simulink model "RealTimeMachine"  (R2021a)
settings: Solver=FixedStepDiscrete  StartTime=0.0  StopTime=Inf  FixedStep=TSampleRTM  MaxStep=1e-3  RelTol=1e-3  EnableMultiTasking=on
settings Model: SimulationMode=external  ExtModeTrigDuration=8  Creator=lu  LastModifiedBy=lu
settings SolverCC: AlgebraicLoopSolver=TrustRegion  AutoInsertRateTranBlk=on
settings OptimizationCC: DefaultUnderspecifiedDataType=single  PassReuseOutputArgsAs=Individual arguments  MaxStackSize=1024  DenormalBehavior=FlushToZero  EfficientTunableParamExpr=on
settings DebuggingCC: ParameterTunabilityLossMsg=error  SFMachineParentedDataDiag=warning
settings HardwareCC: ProdBitPerChar=16  ProdBitPerInt=16  ProdBitPerPointer=32  ProdBitPerSizeT=32  ProdBitPerPtrDiffT=32  ProdLargestAtomicInteger=Integer  ProdLargestAtomicFloat=None  ProdWordSize=16  ProdLongLongMode=on  ProdHWDeviceType=Texas Instruments->C2000
settings ModelReferenceCC: ModelReferenceNumInstancesAllowed=Single
settings SFSimCC: MATLABDynamicMemAlloc=off
settings RTWCC: SystemTargetFile=ert.tlc  HardwareBoard=TI Piccolo F28004x  GenCodeOnly=on  TemplateMakefile=ert_default_tmf  GenerateReport=on  Toolchain=Texas Instruments Code Composer Studio (C2000)  IncludeHyperlinkInReport=on  LaunchReport=on  GenerateTraceInfo=on  GenerateTraceReport=on  GenerateTraceReportSl=on  GenerateTraceReportSf=on  GenerateTraceReportEml=on  GenerateWebview=on  GenerateCodeMetricsReport=on
settings CodeAppCC: ForceParamTrailComments=on  IgnoreCustomStorageClasses=off  OperatorAnnotations=on  SimulinkDataObjDesc=on  SFDataObjDesc=on  MATLABFcnDesc=on  InsertBlockDesc=on  StateflowObjectComments=on  MATLABSourceComments=on
settings ERTTargetCC: CodeReplacementLibrary=TI C28x  IncludeMdlTerminateFcn=off  SuppressErrorStatus=on  ExtModeTransport=3  ExtModeStaticAllocSize=5000

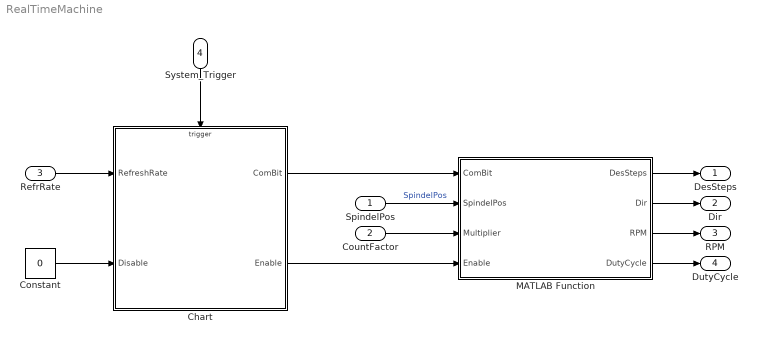
== system RealTimeMachine ==
  SpindelPos : Inport  OutDataTypeStr=uint32
  CountFactor : Inport  Port=2  OutDataTypeStr=double
  RefrRate : Inport  Port=3  OutDataTypeStr=uint16
  System_Trigger : Inport  Port=4  OutDataTypeStr=uint8
  Chart : Stateflow chart  TreatAsAtomicUnit=on
  Constant : Constant  Value=0  OutDataTypeStr=uint16
  MATLAB Function : MATLAB Function  TreatAsAtomicUnit=on
  DesSteps : Outport  OutDataTypeStr=uint16
  Dir : Outport  Port=2  OutDataTypeStr=uint16
  RPM : Outport  Port=3  OutDataTypeStr=uint16
  DutyCycle : Outport  Port=4  OutDataTypeStr=uint16
  wires:
  System_Trigger/1 -> Chart/Trigger
  MATLAB Function/1(DesSteps) -> DesSteps/1
  CountFactor/1 -> MATLAB Function/3(Multiplier)
  SpindelPos/1 -> MATLAB Function/2(SpindelPos)  "SpindelPos"
  RefrRate/1 -> Chart/1(RefreshRate)
  MATLAB Function/3(RPM) -> RPM/1
  MATLAB Function/4(DutyCycle) -> DutyCycle/1
  MATLAB Function/2(Dir) -> Dir/1
  Constant/1 -> Chart/2(Disable)
  Chart/2(Enable) -> MATLAB Function/4(Enable)
  Chart/1(ComBit) -> MATLAB Function/1(ComBit)

== matlab function RealTimeMachine/MATLAB Function ==
  data: ComBit input; SpindelPos input; Multiplier input; Enable input; DesSteps output; Dir output; RPM output; DutyCycle output
function [DesSteps, Dir, RPM, DutyCycle] = fcn(ComBit, SpindelPos, Multiplier, Enable)

% Initialization of Variables and Outputs
RPM = uint16(0);
DutyCycle = uint16(130);
Dir = uint16(0);
DesSteps = uint16(0);

%% Declaration of constants
TotalStepTime = uint16(80); %Total time a pulse train is allowed to take in us
rpmRefreshRate = uint16(1000); %RPM calculation Frequency
SingleStepDC = uint16(4); %Single Step Dutycycle in 3us clock cycles (x*3us high, x*3us low)
MaxPos = 0x00FFFFFF; %Point on which the encoder register will overflow 


%% Declaration of persistant variables
persistent Carrier
persistent rpmSteps
persistent PrevSpindelpos

if isempty(Carrier)
    Carrier = 0;
end 

if isempty(rpmSteps)
    rpmSteps = uint32(0);
end

if isempty(PrevSpindelpos)
    PrevSpindelpos = uint32(0);
end

if (SpindelPos ~= PrevSpindelpos) && Enable
    % Spindel in motion
    %% Deal with encoder over/underflow and determine direction
    
    if (SpindelPos > PrevSpindelpos) && ((SpindelPos - PrevSpindelpos) > (MaxPos/2))
        SpindelDiv = (MaxPos - SpindelPos) + PrevSpindelpos;
        PrevSpindelpos = SpindelPos;
        Dir = uint16(0);
        
    elseif(SpindelPos < PrevSpindelpos) && ((PrevSpindelpos - SpindelPos) > (MaxPos/2))
        SpindelDiv = (MaxPos - PrevSpindelpos) + SpindelPos;
        PrevSpindelpos = SpindelPos;
        Dir = uint16(1);
        
    elseif(SpindelPos < PrevSpindelpos)
        SpindelDiv = (PrevSpindelpos - SpindelPos);
        PrevSpindelpos = SpindelPos;
        Dir = uint16(0);
        
    elseif(SpindelPos > PrevSpindelpos)
        SpindelDiv = SpindelPos - PrevSpindelpos;
        PrevSpindelpos = SpindelPos;
        Dir = uint16(1);
    else
        SpindelDiv = uint32(0);
    end

    %% Calculate Desired Steps
    rpmSteps = rpmSteps + uint32(SpindelDiv);
    Carrier = Carrier + (Multiplier * double(SpindelDiv));
    DesSteps = uint16(floor(Carrier));
    Carrier = Carrier - floor(Carrier);

    %% Calculate Dutycycle
    if DesSteps <= 1
        DutyCycle = uint16(SingleStepDC);
    elseif (TotalStepTime/DesSteps) < 7
        DutyCycle = uint16(2);
    else
        DutyCycle = uint16(((TotalStepTime/DesSteps)/10));
    end
            


    %% Calculate current RPM
    if ComBit
        RPM = uint16((rpmSteps*60*uint32(rpmRefreshRate))/4096);
        rpmSteps = uint32(0);
    end

else
    %% Spindel not moving
    PrevSpindelpos = SpindelPos;
    DutyCycle = uint16(SingleStepDC);
    RPM = uint16(0);
    Dir = uint16(0);
    DesSteps = uint16(0);
end
end

== stateflow chart RealTimeMachine/Chart ==
  settings: sampleTime=100e-6
  state Reset
    Enable = 0;
    ComBit = 0;
  state Main
    state MachineStatus [parallel]
      settings: executionOrder=1
      state Enabled
        en: Enable = 1;
      state Disabled
        en: Enable = 0;
      (default) -> Enabled
      Enabled -> Disabled : [Disable == 1]
      Disabled -> Enabled : [Disable == 0]
    state Communication [parallel]
      settings: executionOrder=2
      state RX
        en: ComBit = 0;
      state TX
        en: ComBit = 1;
      (default) -> RX
      TX -> RX : [after(2,Takt)]
      RX -> TX : [after(RefreshRate,Takt)]
  (default) -> Reset
  Reset -> Main : POR
  data: ComBit output uint16; Enable output uint16; RefreshRate input uint16; Disable input uint16
  events: Takt input EITHER_EDGE_EVENT; POR input RISING_EDGE_EVENT
